simulink model "sim_flexible_unsteady_indi"  (R2018b)
settings: Solver=ode4  StartTime=0.0  StopTime=1000  FixedStep=1/600  RelTol=1e-2  AbsTol=1e-2
model workspace (MAT data in the model file):
  Var = 0
undefined symbols (not defined in the file): aircraft, gla_indi, jystck
libraries: se2a_controller_lib x2, InputBlocks_library x2, se2a_environment_lib x1, flight_dynamics_models x1, sensors_lib x1, aeroelasticity_lib x1, se2a_command_lib x1, joystick_lib x1, dspnetwork x1, flexiFlightVis_lib x1
settings Model: PacingRate=0.100000  ParamWorkspaceSource=ReferencedWorkspace  TunableVars=test_val  TunableVarsStorageClass=ExportedGlobal  Creator=Yannic  LastModifiedBy=yannic
settings DataIOCC: ExternalInput=[0,tp_indi.Input']  InitialState=tp_indi.State  LoadExternalInput=on  LoadInitialState=on
settings DebuggingCC: InitInArrayFormatMsg=none

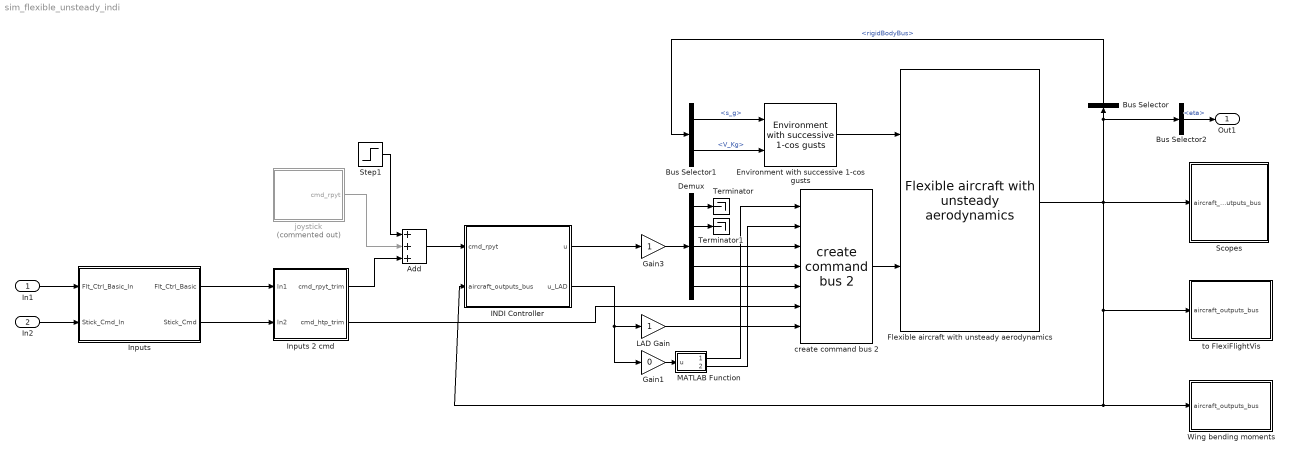
== system sim_flexible_unsteady_indi ==
  In1 : Inport
  In2 : Inport  Port=2
  Add : Sum  Inputs=+++
  Bus Selector : BusSelector  OutputSignals=flexible_body_bus.rigidBodyBus
  Bus Selector1 : BusSelector  OutputSignals=s_g,V_Kg
  Bus Selector2 : BusSelector  OutputSignals=flexible_body_bus.eta
  Demux : Demux  Outputs=5
  Environment with successive 1-cos gusts : se2a_environment_lib/Environment with successive 1-cos gusts  envir=envir  wind_input=2  F_g=1  gustGradDist=100  Delta_gustGradDist=100  Delta_time=3  time_0=1
      settings: SourceProductName=SE2A library
  Flexible aircraft with unsteady aerodynamics : flight_dynamics_models/Flexible aircraft with unsteady aerodynamics  aircraft=aircraft  ic=ic
      settings: SourceProductName=SE2A library
  Gain1 : Gain  Gain=0
  Gain3 : Gain
  INDI Controller : Subsystem
  Inputs : Subsystem
  Inputs 2 cmd : Subsystem
  LAD Gain : Gain
  MATLAB Function : MATLAB Function  TreatAsAtomicUnit=on
  Scopes : Subsystem
  Step1 : Step  Before=zeros(4,1)  After=[0;0.05;0;0]*0  SampleTime=0
  Terminator : Terminator
  Terminator1 : Terminator
  Wing bending moments : Subsystem
  create command bus 2 : se2a_command_lib/create command bus 2
      settings: SourceProductName=SE2A library
  joystick : Subsystem  Commented=on
  to FlexiFlightVis : Subsystem
  Out1 : Outport
  wires:
  Environment with successive 1-cos gusts/1 -> Flexible aircraft with unsteady aerodynamics/1
  create command bus 2/1 -> Flexible aircraft with unsteady aerodynamics/2
  Bus Selector1/1 -> Environment with successive 1-cos gusts/1  "<s_g>"
  Bus Selector/1 -> Bus Selector1/1  "<rigidBodyBus>"
  Bus Selector1/2 -> Environment with successive 1-cos gusts/2  "<V_Kg>"
  joystick/1(cmd_rpyt) -> Add/2
  Flexible aircraft with unsteady aerodynamics/1 -> to FlexiFlightVis/1(aircraft_outputs_bus), Wing bending moments/1(aircraft_outputs_bus), INDI Controller/2(aircraft_outputs_bus), Scopes/1(aircraft_outputs_bus), Bus Selector2/1, Bus Selector/1
  Demux/3 -> create command bus 2/3
  Demux/4 -> create command bus 2/4
  Demux/5 -> create command bus 2/5
  Inputs 2 cmd/2(cmd_htp_trim) -> create command bus 2/6
  In1/1 -> Inputs/1(Flt_Ctrl_Basic_In)
  In2/1 -> Inputs/2(Stick_Cmd_In)
  Inputs/1(Flt_Ctrl_Basic) -> Inputs 2 cmd/1(In1)
  Inputs/2(Stick_Cmd) -> Inputs 2 cmd/2(In2)
  Add/1 -> INDI Controller/1(cmd_rpyt)
  Inputs 2 cmd/1(cmd_rpyt_trim) -> Add/3
  INDI Controller/1(u) -> Gain3/1
  Gain3/1 -> Demux/1
  INDI Controller/2(u_LAD) -> Gain1/1, LAD Gain/1
  Step1/1 -> Add/1
  LAD Gain/1 -> create command bus 2/7
  Bus Selector2/1 -> Out1/1  "<eta>"
  Gain1/1 -> MATLAB Function/1(u)
  MATLAB Function/1(a_l) -> create command bus 2/1
  MATLAB Function/2(a_r) -> create command bus 2/2
  Demux/1 -> Terminator/1
  Demux/2 -> Terminator1/1

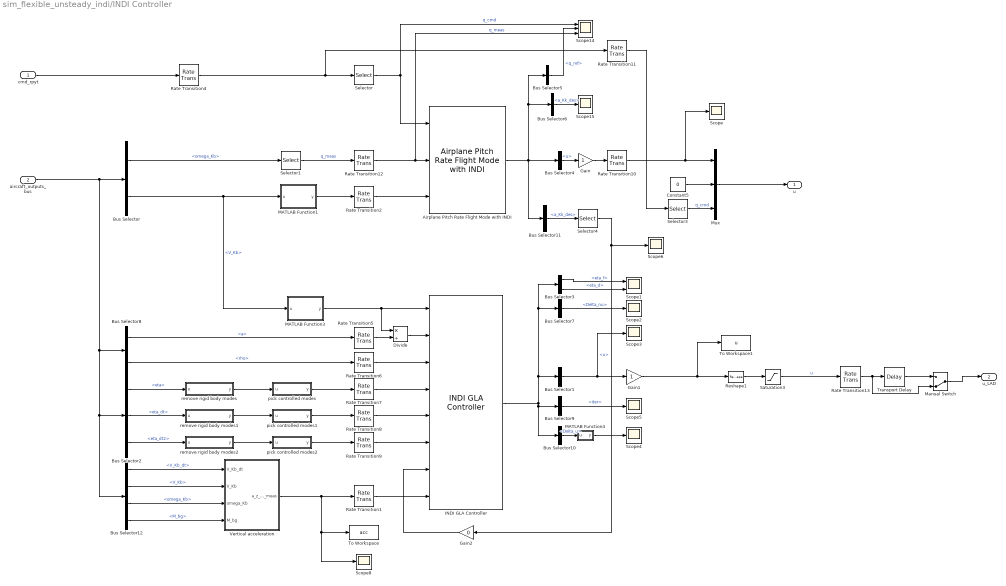
== system sim_flexible_unsteady_indi/INDI Controller ==
  cmd_rpyt : Inport
  aircraft_outputs_bus : Inport  Port=2
  Airplane Pitch Rate Flight Mode with INDI : se2a_controller_lib/Airplane Pitch Rate Flight Mode with INDI  fm=pitch_rate_controller
  Bus Selector : BusSelector  OutputSignals=flexible_body_bus.rigidBodyBus.omega_Kb,flexible_body_bus.rigidBodyBus.V_Kb
  Bus Selector1 : BusSelector  OutputSignals=u
  Bus Selector10 : BusSelector  OutputSignals=Delta_u
  Bus Selector11 : BusSelector  OutputSignals=direct_lift_control.a_Kk_des
  Bus Selector12 : BusSelector  OutputSignals=flexible_body_bus.rigidBodyBus.V_Kb_dt,flexible_body_bus.rigidBodyBus.V_Kb,flexible_body_bus.rigidBodyBus.omega_Kb,flexible_body_bus.rigidBodyBus.M_bg
  Bus Selector2 : BusSelector  OutputSignals=flexible_body_bus.eta,flexible_body_bus.eta_dt,flexible_body_bus.eta_dt2
  Bus Selector3 : BusSelector  OutputSignals=measure.eta_f,desired.eta_d
  Bus Selector4 : BusSelector  OutputSignals=u
  Bus Selector5 : BusSelector  OutputSignals=pitch_rate_control.reference.q_ref
  Bus Selector6 : BusSelector  OutputSignals=direct_lift_control.a_Kk_des
  Bus Selector7 : BusSelector  OutputSignals=pseudo_cntrl.Delta_nu
  Bus Selector8 : BusSelector  OutputSignals=aeroBus.main.external.atmosphere.a,aeroBus.main.external.atmosphere.rho
  Bus Selector9 : BusSelector  OutputSignals=iter
  Constant5 : Constant  Value=0
  Divide : Product  Inputs=*/
  Gain : Gain
  Gain1 : Gain
  Gain2 : Gain  Gain=0
  INDI GLA Controller : se2a_controller_lib/INDI GLA Controller  gla_indi=gla_indi
  MATLAB Function1 : MATLAB Function  TreatAsAtomicUnit=on
  MATLAB Function3 : MATLAB Function  TreatAsAtomicUnit=on
  MATLAB Function4 : MATLAB Function  TreatAsAtomicUnit=on
  Manual Switch : ManualSwitch  CurrentSetting=0
  Mux : Mux  Inputs=3
  Rate Transition{1,5..9} (6 alike) : RateTransition  OutPortSampleTime=gla_indi.ts
  Rate Transition{2,4,10..13} (6 alike) : RateTransition
  Reshape1 : Reshape
  Saturation3 : Saturate  UpperLimit=gla_indi.ca.u_max  LowerLimit=gla_indi.ca.u_min
  Scope{,2..6,8,15} (8 alike) : Scope
  Scope1 : Scope  NumInputPorts=2
  Scope14 : Scope  NumInputPorts=3
  Selector : Selector  InputPortWidth=4  IndexOptions=Index vector (dialog)  Indices=2  OutputSizes=1
  Selector1 : Selector  InputPortWidth=3  IndexOptions=Index vector (dialog)  Indices=2  OutputSizes=1
  Selector3 : Selector  InputPortWidth=4  IndexOptions=Index vector (dialog)  Indices=4  OutputSizes=1
  Selector4 : Selector  InputPortWidth=3  IndexOptions=Index vector (dialog)  Indices=3  OutputSizes=1
  To Workspace : ToWorkspace  VariableName=acc  SaveFormat=Timeseries  SampleTime=-1
  To Workspace1 : ToWorkspace  VariableName=u  SaveFormat=Timeseries  SampleTime=-1
  Transport Delay : TransportDelay  DelayTime=gla_indi.ts  TransDelayFeedthrough=on
  Vertical acceleration : Subsystem
  pick controlled modes : MATLAB Function  TreatAsAtomicUnit=on
  pick controlled modes1 : MATLAB Function  TreatAsAtomicUnit=on
  pick controlled modes2 : MATLAB Function  TreatAsAtomicUnit=on
  remove rigid body modes : MATLAB Function  TreatAsAtomicUnit=on
  remove rigid body modes1 : MATLAB Function  TreatAsAtomicUnit=on
  remove rigid body modes2 : MATLAB Function  TreatAsAtomicUnit=on
  u : Outport
  u_LAD : Outport  Port=2
  wires:
  cmd_rpyt/1 -> Rate Transition4/1
  aircraft_outputs_bus/1 -> Bus Selector12/1, Bus Selector2/1, Bus Selector8/1, Bus Selector/1
  Bus Selector/1 -> Selector1/1  "<omega_Kb>"
  Bus Selector/2 -> MATLAB Function3/1(u), MATLAB Function1/1(u)  "<V_Kb>"
  Rate Transition2/1 -> Airplane Pitch Rate Flight Mode with INDI/3
  Rate Transition4/1 -> Rate Transition11/1, Selector/1
  Bus Selector4/1 -> Gain/1  "<u>"
  Rate Transition10/1 -> Scope/1, Mux/1
  Constant5/1 -> Mux/2
  Bus Selector5/1 -> Scope14/2  "<q_ref>"
  Selector/1 -> Airplane Pitch Rate Flight Mode with INDI/1, Scope14/1  "q_cmd"
  Bus Selector6/1 -> Scope15/1  "<a_Kk_des>"
  Rate Transition12/1 -> Airplane Pitch Rate Flight Mode with INDI/2, Scope14/3  "q_meas"
  Airplane Pitch Rate Flight Mode with INDI/1 -> Bus Selector5/1, Bus Selector6/1, Bus Selector11/1, Bus Selector4/1
  Mux/1 -> u/1
  Bus Selector2/1 -> remove rigid body modes/1(u)  "<eta>"
  INDI GLA Controller/1 -> Bus Selector10/1, Bus Selector9/1, Bus Selector7/1, Bus Selector3/1, Bus Selector1/1
  Bus Selector2/2 -> remove rigid body modes1/1(u)  "<eta_dt>"
  Bus Selector2/3 -> remove rigid body modes2/1(u)  "<eta_dt2>"
  Bus Selector1/1 -> Scope3/1, Gain1/1  "<u>"
  Bus Selector3/1 -> Scope1/1  "<eta_f>"
  Bus Selector3/2 -> Scope1/2  "<eta_d>"
  Gain/1 -> Rate Transition10/1
  remove rigid body modes/1(y) -> pick controlled modes/1(u)
  remove rigid body modes1/1(y) -> pick controlled modes1/1(u)
  remove rigid body modes2/1(y) -> pick controlled modes2/1(u)
  Bus Selector7/1 -> Scope2/1  "<Delta_nu>"
  Bus Selector8/2 -> Rate Transition6/1  "<rho>"
  Bus Selector8/1 -> Rate Transition5/1  "<a>"
  Bus Selector9/1 -> Scope5/1  "<iter>"
  Divide/1 -> INDI GLA Controller/2
  Rate Transition5/1 -> Divide/2
  Rate Transition6/1 -> INDI GLA Controller/3
  Rate Transition7/1 -> INDI GLA Controller/4
  Rate Transition8/1 -> INDI GLA Controller/5
  Rate Transition9/1 -> INDI GLA Controller/6
  Selector3/1 -> Mux/3  "q_cmd"
  Rate Transition11/1 -> Selector3/1
  Rate Transition13/1 -> Manual Switch/2, Transport Delay/1
  Gain1/1 -> To Workspace1/1, Reshape1/1
  Transport Delay/1 -> Manual Switch/1
  Reshape1/1 -> Saturation3/1
  Bus Selector10/1 -> MATLAB Function4/1(u)  "<Delta_u>"
  MATLAB Function4/1(y) -> Scope4/1
  Saturation3/1 -> Rate Transition13/1  "u"
  Bus Selector11/1 -> Selector4/1  "<a_Kk_des>"
  Selector4/1 -> Scope6/1, Gain2/1
  pick controlled modes/1(y) -> Rate Transition7/1
  pick controlled modes1/1(y) -> Rate Transition8/1
  pick controlled modes2/1(y) -> Rate Transition9/1
  Manual Switch/1 -> u_LAD/1
  Selector1/1 -> Rate Transition12/1  "q_meas"
  MATLAB Function3/1(y) -> INDI GLA Controller/1, Divide/1
  Gain2/1 -> INDI GLA Controller/7
  MATLAB Function1/1(y) -> Rate Transition2/1
  Bus Selector12/1 -> Vertical acceleration/1(V_Kb_dt)  "<V_Kb_dt>"
  Bus Selector12/2 -> Vertical acceleration/2(V_Kb)  "<V_Kb>"
  Bus Selector12/3 -> Vertical acceleration/3(omega_Kb)  "<omega_Kb>"
  Bus Selector12/4 -> Vertical acceleration/4(M_bg)  "<M_bg>"
  Vertical acceleration/1(a_z_Kb_meas) -> Scope8/1, To Workspace/1, Rate Transition1/1
  Rate Transition1/1 -> INDI GLA Controller/8

== system sim_flexible_unsteady_indi/Inputs ==
  Flt_Ctrl_Basic_In : Inport
  Stick_Cmd_In : Inport  Port=2
  FltCtrlBasic : InputBlocks_library/FltCtrlBasic  SystemSampleTime=-1
  StickCmd : InputBlocks_library/StickCmd  SystemSampleTime=-1
  Flt_Ctrl_Basic : Outport
  Stick_Cmd : Outport  Port=2
  wires:
  StickCmd/1 -> Stick_Cmd/1
  FltCtrlBasic/1 -> Flt_Ctrl_Basic/1
  Flt_Ctrl_Basic_In/1 -> FltCtrlBasic/1
  Stick_Cmd_In/1 -> StickCmd/1

== system sim_flexible_unsteady_indi/Inputs 2 cmd ==
  In1 : Inport
  In2 : Inport  Port=2
  Demux : Demux  Outputs=2
  Mux : Mux  Inputs=2
  Selector : Selector  InputPortWidth=4  IndexOptions=Index vector (dialog)  Indices=1:3  OutputSizes=1
  cmd_rpyt_trim : Outport
  cmd_htp_trim : Outport  Port=2
  wires:
  Demux/1 -> Mux/2
  Selector/1 -> Mux/1
  Mux/1 -> cmd_rpyt_trim/1
  In1/1 -> Demux/1
  Demux/2 -> cmd_htp_trim/1
  In2/1 -> Selector/1

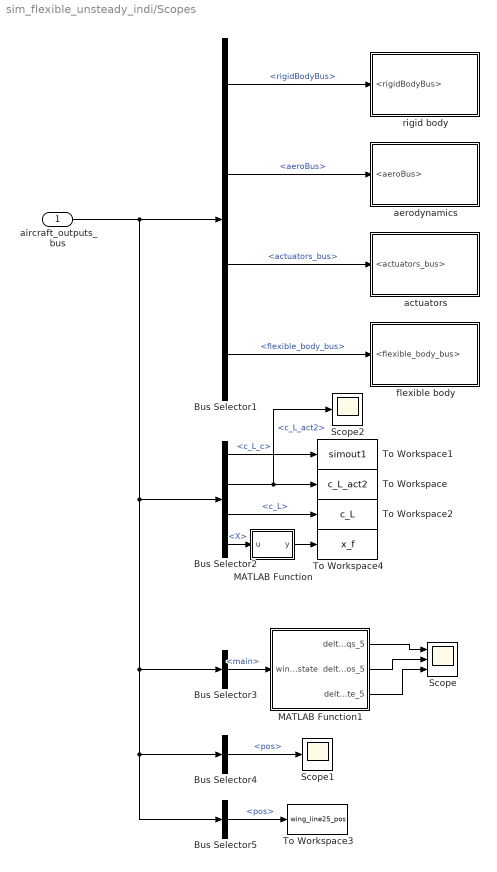
== system sim_flexible_unsteady_indi/Scopes ==
  aircraft_outputs_bus : Inport
  Bus Selector1 : BusSelector  OutputSignals=flexible_body_bus.rigidBodyBus,aeroBus,actuators_bus,flexible_body_bus
  Bus Selector2 : BusSelector  OutputSignals=aeroBus.main.aero.unsteady.c_L_c,aeroBus.main.aero.unsteady.c_L_act2,aeroBus.main.aero.circulation.c_L,aeroBus.main.aero.unsteady.X
  Bus Selector3 : BusSelector  OutputSignals=aeroBus.main
  Bus Selector4 : BusSelector  OutputSignals=aeroBus.main.actuators.pos
  Bus Selector5 : BusSelector  OutputSignals=aeroBus.main.geometry.line_25.pos
  MATLAB Function : MATLAB Function  TreatAsAtomicUnit=on
  MATLAB Function1 : MATLAB Function  TreatAsAtomicUnit=on
  Scope : Scope  NumInputPorts=3
  Scope1 : Scope
  Scope2 : Scope
  To Workspace : ToWorkspace  VariableName=c_L_act2  SaveFormat=Timeseries  SampleTime=-1
  To Workspace1 : ToWorkspace  VariableName=simout1  SaveFormat=Timeseries  SampleTime=-1
  To Workspace2 : ToWorkspace  VariableName=c_L  SaveFormat=Timeseries  SampleTime=-1
  To Workspace3 : ToWorkspace  VariableName=wing_line25_pos  SaveFormat=Timeseries  SampleTime=-1
  To Workspace4 : ToWorkspace  VariableName=x_f  SaveFormat=Timeseries  SampleTime=-1
  actuators : Subsystem
  aerodynamics : Subsystem
  flexible body : Subsystem
  rigid body : Subsystem
  wires:
  Bus Selector1/1 -> rigid body/1(<rigidBodyBus>)  "<rigidBodyBus>"
  Bus Selector1/2 -> aerodynamics/1(<aeroBus>)  "<aeroBus>"
  Bus Selector1/3 -> actuators/1(<actuators_bus>)  "<actuators_bus>"
  Bus Selector1/4 -> flexible body/1(<flexible_body_bus>)  "<flexible_body_bus>"
  MATLAB Function1/1(delta_qs_5) -> Scope/1
  MATLAB Function1/3(delta_qs_rate_5) -> Scope/3
  Bus Selector2/3 -> To Workspace2/1  "<c_L>"
  MATLAB Function1/2(delta_qs_pos_5) -> Scope/2
  Bus Selector3/1 -> MATLAB Function1/1(wing_state)  "<main>"
  Bus Selector2/2 -> Scope2/1, To Workspace/1  "<c_L_act2>"
  aircraft_outputs_bus/1 -> Bus Selector5/1, Bus Selector4/1, Bus Selector3/1, Bus Selector2/1, Bus Selector1/1
  Bus Selector2/1 -> To Workspace1/1  "<c_L_c>"
  Bus Selector4/1 -> Scope1/1  "<pos>"
  Bus Selector5/1 -> To Workspace3/1  "<pos>"
  Bus Selector2/4 -> MATLAB Function/1(u)  "<X>"
  MATLAB Function/1(y) -> To Workspace4/1

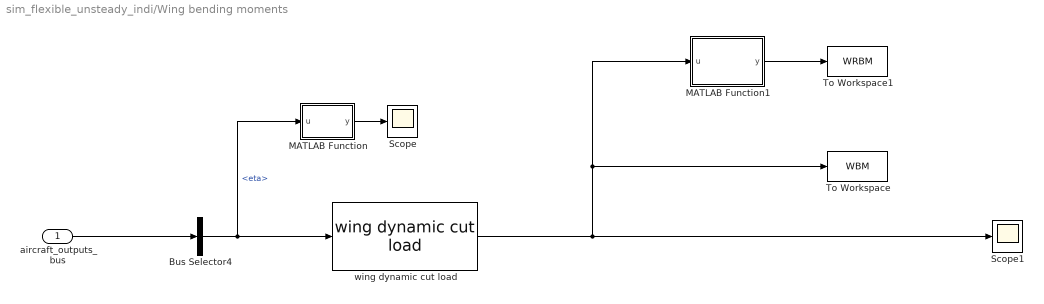
== system sim_flexible_unsteady_indi/Wing bending moments ==
  aircraft_outputs_bus : Inport
  Bus Selector4 : BusSelector  OutputSignals=flexible_body_bus.eta
  MATLAB Function : MATLAB Function  TreatAsAtomicUnit=on
  MATLAB Function1 : MATLAB Function  TreatAsAtomicUnit=on
  Scope : Scope
  Scope1 : Scope
  To Workspace : ToWorkspace  VariableName=WBM  SaveFormat=Timeseries  SampleTime=-1
  To Workspace1 : ToWorkspace  VariableName=WRBM  SaveFormat=Timeseries  SampleTime=-1
  wing dynamic cut load : aeroelasticity_lib/wing dynamic cut load  structure=structure  structure_red=aircraft.eom_flexible.structure_red  eta=[-0.9:0.2:0.9]  popup_index_1=Mx  popup_index_2=reverse_right
      settings: SourceProductName=LADAC
  wires:
  Bus Selector4/1 -> wing dynamic cut load/1, MATLAB Function/1(u)  "<eta>"
  aircraft_outputs_bus/1 -> Bus Selector4/1
  wing dynamic cut load/1 -> Scope1/1, To Workspace/1, MATLAB Function1/1(u)
  MATLAB Function/1(y) -> Scope/1
  MATLAB Function1/1(y) -> To Workspace1/1

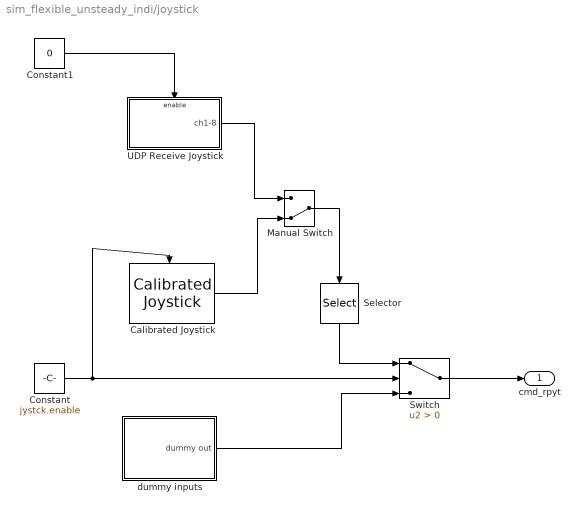
== system sim_flexible_unsteady_indi/joystick ==
  Calibrated Joystick : joystick_lib/Calibrated Joystick  jystck=jystck
      settings: SourceProductName=LADAC
  Constant : Constant  Value=jystck.enable
  Constant1 : Constant  Value=0
  Manual Switch : ManualSwitch  CurrentSetting=0
  Selector : Selector  InputPortWidth=8  IndexOptions=Index vector (dialog)  Indices=[1,2,3,4]  OutputSizes=1
  Switch : Switch  Criteria=u2 > Threshold
  UDP Receive Joystick : Subsystem
  dummy inputs : Subsystem
  cmd_rpyt : Outport
  wires:
  Switch/1 -> cmd_rpyt/1
  Constant/1 -> Calibrated Joystick/Enable, Switch/2
  dummy inputs/1(dummy out) -> Switch/3
  Selector/1 -> Switch/1
  UDP Receive Joystick/1(ch1-8) -> Manual Switch/1
  Manual Switch/1 -> Selector/1
  Calibrated Joystick/1 -> Manual Switch/2
  Constant1/1 -> UDP Receive Joystick/Enable

== system sim_flexible_unsteady_indi/to FlexiFlightVis ==
  aircraft_outputs_bus : Inport
  Bus Creator : BusCreator  Inputs=1
  Bus Selector : BusSelector  OutputSignals=flexible_body_bus.rigidBodyBus,aeroBus.main,aeroBus.htp,aeroBus.vtp,aeroBus.fuselage
  Constant : Constant  Value=aircraft.config.xyz_ref_c
  Send to FlexiFlightVis : flexiFlightVis_lib/Send to FlexiFlightVis  sample_time=1/60  ip_address='localhost'  ip_port=4321  wing_cell={aircraft.wing_main.state,aircraft.wing_htp.state,aircraft.wing_vtp.state}  fuse_cell={aircraft.fuselage.state}
      settings: SourceProductName=LADAC
  wires:
  aircraft_outputs_bus/1 -> Bus Selector/1
  Bus Selector/4 -> Send to FlexiFlightVis/5  "<vtp>"
  Bus Selector/5 -> Send to FlexiFlightVis/6  "<fuselage>"
  Bus Selector/3 -> Send to FlexiFlightVis/4  "<htp>"
  Bus Selector/2 -> Send to FlexiFlightVis/3  "<main>"
  Bus Selector/1 -> Send to FlexiFlightVis/1  "<rigidBodyBus>"
  Constant/1 -> Bus Creator/1  "xyz_ref_c"
  Bus Creator/1 -> Send to FlexiFlightVis/2

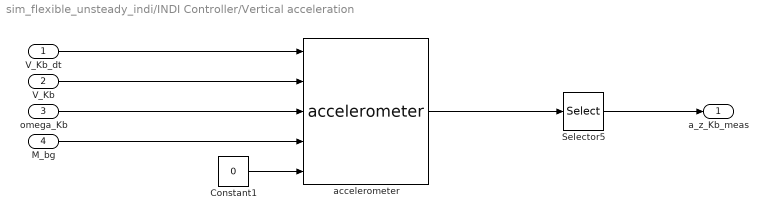
== system sim_flexible_unsteady_indi/INDI Controller/Vertical acceleration ==
  V_Kb_dt : Inport
  V_Kb : Inport  Port=2
  omega_Kb : Inport  Port=3
  M_bg : Inport  Port=4
  Constant1 : Constant  Value=0  VectorParams1D=off
  Selector5 : Selector  InputPortWidth=3  IndexOptions=Index vector (dialog)  Indices=3  OutputSizes=1
  accelerometer : sensors_lib/accelerometer  SystemSampleTime=-1
      settings: SourceProductName=LADAC
  a_z_Kb_meas : Outport
  wires:
  M_bg/1 -> accelerometer/4
  Selector5/1 -> a_z_Kb_meas/1
  accelerometer/1 -> Selector5/1
  V_Kb/1 -> accelerometer/2
  omega_Kb/1 -> accelerometer/3
  V_Kb_dt/1 -> accelerometer/1
  Constant1/1 -> accelerometer/5

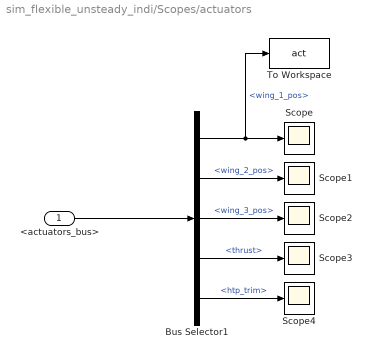
== system sim_flexible_unsteady_indi/Scopes/actuators ==
  <actuators_bus> : Inport
  Bus Selector1 : BusSelector  OutputSignals=wing_1_pos,wing_2_pos,wing_3_pos,thrust,htp_trim
  Scope{,1..4} (5 alike) : Scope
  To Workspace : ToWorkspace  VariableName=act  SaveFormat=Timeseries  SampleTime=-1
  wires:
  <actuators_bus>/1 -> Bus Selector1/1
  Bus Selector1/1 -> To Workspace/1, Scope/1  "<wing_1_pos>"
  Bus Selector1/2 -> Scope1/1  "<wing_2_pos>"
  Bus Selector1/3 -> Scope2/1  "<wing_3_pos>"
  Bus Selector1/4 -> Scope3/1  "<thrust>"
  Bus Selector1/5 -> Scope4/1  "<htp_trim>"

== system sim_flexible_unsteady_indi/Scopes/aerodynamics ==
  <aeroBus> : Inport
  Bus Selector1 : BusSelector  OutputSignals=main,htp,vtp
  htp : Subsystem
  vtp : Subsystem
  wing : Subsystem
  wires:
  <aeroBus>/1 -> Bus Selector1/1
  Bus Selector1/2 -> htp/1(htp)  "<htp>"
  Bus Selector1/1 -> wing/1(main)  "<main>"
  Bus Selector1/3 -> vtp/1(vtp)  "<vtp>"

== system sim_flexible_unsteady_indi/Scopes/flexible body ==
  <flexible_body_bus> : Inport
  Bus Selector1 : BusSelector  OutputSignals=eta,eta_dt,eta_dt2,generalized_load_vector
  Scope{,1..3} (4 alike) : Scope
  To Workspace : ToWorkspace  VariableName=eta  SaveFormat=Timeseries  SampleTime=-1
  wires:
  Bus Selector1/4 -> Scope3/1  "<generalized_load_vector>"
  Bus Selector1/3 -> Scope2/1  "<eta_dt2>"
  Bus Selector1/2 -> Scope1/1  "<eta_dt>"
  Bus Selector1/1 -> To Workspace/1, Scope/1  "<eta>"
  <flexible_body_bus>/1 -> Bus Selector1/1

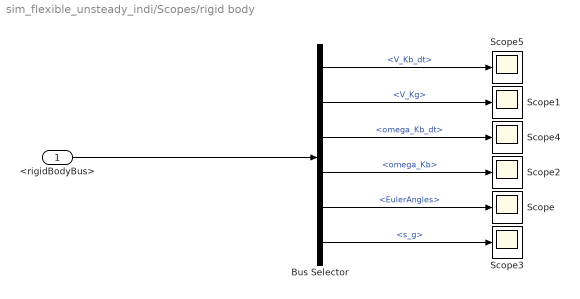
== system sim_flexible_unsteady_indi/Scopes/rigid body ==
  <rigidBodyBus> : Inport
  Bus Selector : BusSelector  OutputSignals=V_Kb_dt,V_Kg,omega_Kb_dt,omega_Kb,EulerAngles,s_g
  Scope{,1..5} (6 alike) : Scope
  wires:
  Bus Selector/5 -> Scope/1  "<EulerAngles>"
  Bus Selector/2 -> Scope1/1  "<V_Kg>"
  Bus Selector/6 -> Scope3/1  "<s_g>"
  Bus Selector/4 -> Scope2/1  "<omega_Kb>"
  <rigidBodyBus>/1 -> Bus Selector/1
  Bus Selector/3 -> Scope4/1  "<omega_Kb_dt>"
  Bus Selector/1 -> Scope5/1  "<V_Kb_dt>"

== system sim_flexible_unsteady_indi/joystick/UDP Receive Joystick ==
  Enable : EnablePort
  Terminator : Terminator
  UDP Receive1 : dspnetwork/UDP Receive  localURL='0.0.0.0'  localPort=25000  remoteURL='192.168.178.2'  remotePort=-1  recvBufferSize=8*8  dims=8  signalDatatype=double  isVarSize=off  showBlockingTime=on  blockingTime=1  sampletime=1/30  blockPlatform=HOST
      settings: SourceProductName=DSP System Toolbox  SourceProductBaseCode=DS
  ch1-8 : Outport
  wires:
  UDP Receive1/1 -> ch1-8/1
  UDP Receive1/2 -> Terminator/1

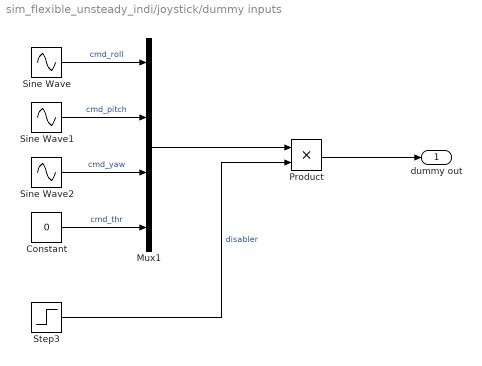
== system sim_flexible_unsteady_indi/joystick/dummy inputs ==
  Constant : Constant  Value=0
  Mux1 : Mux
  Product : Product
  Sine Wave : Sin  Amplitude=0.1  Frequency=3  SampleTime=0
  Sine Wave1 : Sin  Amplitude=0.1  Frequency=4  SampleTime=0
  Sine Wave2 : Sin  Amplitude=0.1  Frequency=5  SampleTime=0
  Step3 : Step  Time=10  Before=1  After=0  SampleTime=0
  dummy out : Outport
  wires:
  Constant/1 -> Mux1/4  "cmd_thr"
  Sine Wave2/1 -> Mux1/3  "cmd_yaw"
  Sine Wave1/1 -> Mux1/2  "cmd_pitch"
  Sine Wave/1 -> Mux1/1  "cmd_roll"
  Mux1/1 -> Product/1
  Product/1 -> dummy out/1
  Step3/1 -> Product/2  "disabler"

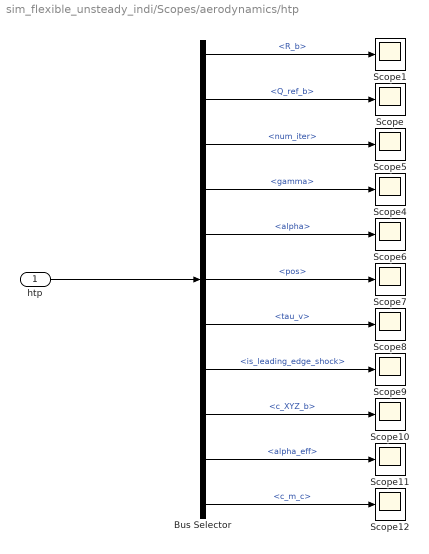
== system sim_flexible_unsteady_indi/Scopes/aerodynamics/htp ==
  htp : Inport
  Bus Selector : BusSelector  OutputSignals=aero.force_glob.R_b,aero.force_glob.Q_ref_b,aero.circulation.num_iter,aero.circulation.gamma,body.alpha,actuators.pos,aero.unsteady.tau_v,aero.unsteady.is_leading_edge_shock,aero.coeff_loc.c_XYZ_b,aero.circulation.alpha_eff,aero.unsteady.c_m_c
  Scope{,1,4..12} (11 alike) : Scope
  wires:
  Bus Selector/11 -> Scope12/1  "<c_m_c>"
  Bus Selector/10 -> Scope11/1  "<alpha_eff>"
  Bus Selector/9 -> Scope10/1  "<c_XYZ_b>"
  Bus Selector/8 -> Scope9/1  "<is_leading_edge_shock>"
  Bus Selector/7 -> Scope8/1  "<tau_v>"
  Bus Selector/6 -> Scope7/1  "<pos>"
  Bus Selector/5 -> Scope6/1  "<alpha>"
  htp/1 -> Bus Selector/1
  Bus Selector/1 -> Scope1/1  "<R_b>"
  Bus Selector/2 -> Scope/1  "<Q_ref_b>"
  Bus Selector/4 -> Scope4/1  "<gamma>"
  Bus Selector/3 -> Scope5/1  "<num_iter>"

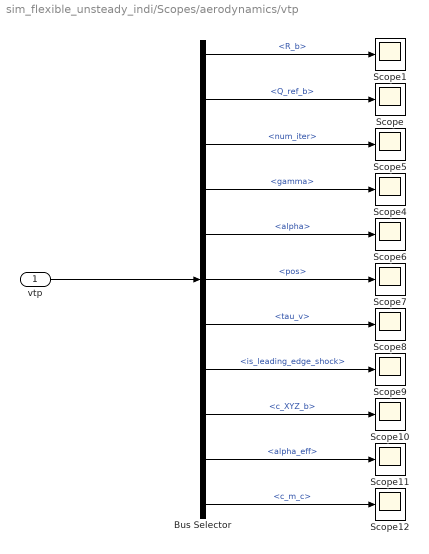
== system sim_flexible_unsteady_indi/Scopes/aerodynamics/vtp ==
  vtp : Inport
  Bus Selector : BusSelector  OutputSignals=aero.force_glob.R_b,aero.force_glob.Q_ref_b,aero.circulation.num_iter,aero.circulation.gamma,body.alpha,actuators.pos,aero.unsteady.tau_v,aero.unsteady.is_leading_edge_shock,aero.coeff_loc.c_XYZ_b,aero.circulation.alpha_eff,aero.unsteady.c_m_c
  Scope{,1,4..12} (11 alike) : Scope
  wires:
  Bus Selector/3 -> Scope5/1  "<num_iter>"
  Bus Selector/4 -> Scope4/1  "<gamma>"
  Bus Selector/2 -> Scope/1  "<Q_ref_b>"
  Bus Selector/1 -> Scope1/1  "<R_b>"
  vtp/1 -> Bus Selector/1
  Bus Selector/5 -> Scope6/1  "<alpha>"
  Bus Selector/6 -> Scope7/1  "<pos>"
  Bus Selector/7 -> Scope8/1  "<tau_v>"
  Bus Selector/8 -> Scope9/1  "<is_leading_edge_shock>"
  Bus Selector/9 -> Scope10/1  "<c_XYZ_b>"
  Bus Selector/10 -> Scope11/1  "<alpha_eff>"
  Bus Selector/11 -> Scope12/1  "<c_m_c>"

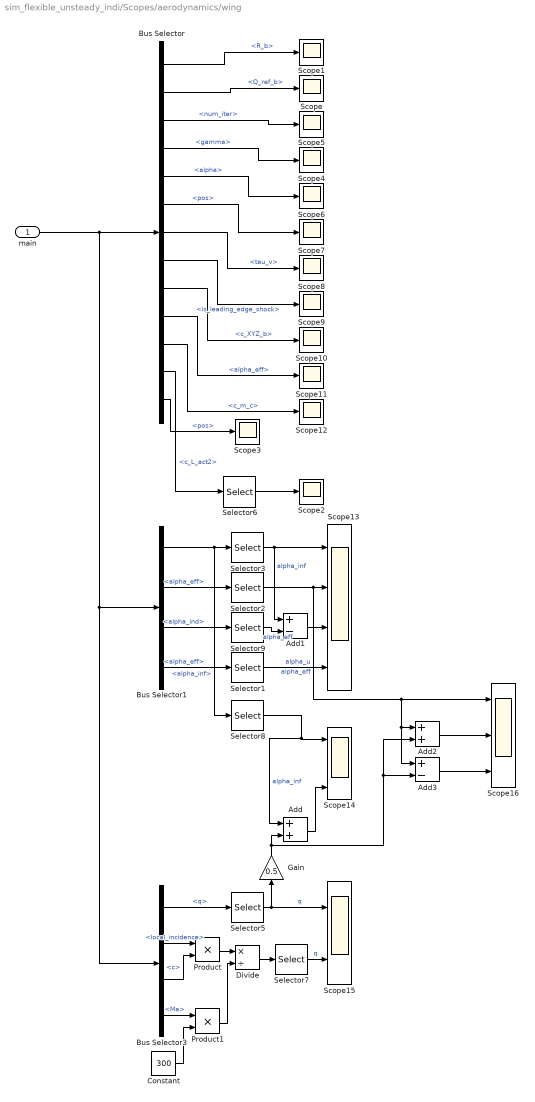
== system sim_flexible_unsteady_indi/Scopes/aerodynamics/wing ==
  main : Inport
  Add : Sum
  Add1 : Sum  Inputs=+-
  Add2 : Sum
  Add3 : Sum  Inputs=+-
  Bus Selector : BusSelector  OutputSignals=aero.force_glob.R_b,aero.force_glob.Q_ref_b,aero.circulation.num_iter,aero.circulation.gamma,body.alpha,actuators.pos,aero.unsteady.tau_v,aero.unsteady.is_leading_edge_shock,aero.coeff_loc.c_XYZ_b,aero.circulation.alpha_eff,aero.unsteady.c_m_c,aero.unsteady.c_L_act2,actuators.pos
  Bus Selector1 : BusSelector  OutputSignals=aero.circulation.alpha_inf,aero.circulation.alpha_eff,aero.circulation.alpha_ind,aero.unsteady.alpha_eff
  Bus Selector3 : BusSelector  OutputSignals=aero.circulation.q,geometry.ctrl_pt_dt.local_incidence,geometry.ctrl_pt.c,aero.circulation.Ma
  Constant : Constant  Value=300
  Divide : Product  Inputs=*/
  Gain : Gain  Gain=0.5
  Product : Product
  Product1 : Product
  Scope{,1..12} (13 alike) : Scope
  Scope13 : Scope  NumInputPorts=4
  Scope14 : Scope  NumInputPorts=3
  Scope15 : Scope  NumInputPorts=2
  Scope16 : Scope  NumInputPorts=3
  Selector{1..3,5,7..9} (7 alike) : Selector  InputPortWidth=40  IndexOptions=Index vector (dialog)  Indices=1:2:9  OutputSizes=1
  Selector6 : Selector  InputPortWidth=40  IndexOptions=Index vector (dialog)  Indices=1:20  OutputSizes=1
  wires:
  Bus Selector/3 -> Scope5/1  "<num_iter>"
  Bus Selector/4 -> Scope4/1  "<gamma>"
  Bus Selector/2 -> Scope/1  "<Q_ref_b>"
  Bus Selector/1 -> Scope1/1  "<R_b>"
  main/1 -> Bus Selector3/1, Bus Selector1/1, Bus Selector/1
  Bus Selector/5 -> Scope6/1  "<alpha>"
  Bus Selector/6 -> Scope7/1  "<pos>"
  Bus Selector/7 -> Scope8/1  "<tau_v>"
  Bus Selector/8 -> Scope9/1  "<is_leading_edge_shock>"
  Bus Selector/9 -> Scope10/1  "<c_XYZ_b>"
  Bus Selector/10 -> Scope11/1  "<alpha_eff>"
  Bus Selector/11 -> Scope12/1  "<c_m_c>"
  Selector6/1 -> Scope2/1
  Bus Selector/12 -> Selector6/1  "<c_L_act2>"
  Bus Selector/13 -> Scope3/1  "<pos>"
  Bus Selector1/1 -> Selector3/1, Selector8/1  "<alpha_inf>"
  Bus Selector1/2 -> Selector2/1  "<alpha_eff>"
  Bus Selector1/4 -> Selector1/1  "<alpha_eff>"
  Selector3/1 -> Add1/1, Scope13/1  "alpha_inf"
  Selector2/1 -> Add3/1, Add2/1, Scope16/1, Scope13/2  "alpha_eff"
  Selector1/1 -> Scope13/4  "alpha_u"
  Bus Selector3/1 -> Selector5/1  "<q>"
  Selector5/1 -> Gain/1, Scope15/1  "q"
  Bus Selector3/2 -> Product/1  "<local_incidence>"
  Bus Selector3/3 -> Product/2  "<c>"
  Product/1 -> Divide/1
  Bus Selector3/4 -> Product1/1  "<Ma>"
  Constant/1 -> Product1/2
  Product1/1 -> Divide/2
  Divide/1 -> Selector7/1
  Selector7/1 -> Scope15/2  "q"
  Gain/1 -> Add2/2, Add3/2, Add/2
  Add/1 -> Scope14/3
  Selector8/1 -> Add/1, Scope14/1  "alpha_inf"
  Bus Selector1/3 -> Selector9/1  "<alpha_ind>"
  Selector9/1 -> Add1/2  "alpha_eff"
  Add1/1 -> Scope13/3
  Add2/1 -> Scope16/2
  Add3/1 -> Scope16/3

== matlab function sim_flexible_unsteady_indi/INDI Controller/pick controlled modes1 ==
  data: u input; y output; gla_indi parameter
function y = fcn(u,gla_indi)
y = u(gla_indi.mcidx);
end

== matlab function sim_flexible_unsteady_indi/INDI Controller/MATLAB Function3 ==
  data: u input; y output
function y = fcn(u)
y=norm(u,2);
end

== matlab function sim_flexible_unsteady_indi/INDI Controller/pick controlled modes2 ==
  data: u input; y output; gla_indi parameter
function y = fcn(u,gla_indi)
y = u(gla_indi.mcidx);
end

== matlab function sim_flexible_unsteady_indi/Scopes/MATLAB Function1 ==
  data: wing_state input; delta_qs_5 output; delta_qs_pos_5 output; delta_qs_rate_5 output
function [delta_qs_5,delta_qs_pos_5,delta_qs_rate_5] = fcn(wing_state)

abs_V_i = vecnorm(wing_state.aero.local_inflow.V_25,2,1);
F = airfoilFlapEffectiveness(wing_state.geometry.segments.flap_depth);
delta_qs = airfoilFlapDeltaQs( F.F_10, F.F_11,...
    abs_V_i, sum(wing_state.geometry.ctrl_pt.c,3), deg2rad(wing_state.actuators.segments.pos(2,:)), ...
    deg2rad(wing_state.actuators.segments.rate(2,:)) ) .* cos(wing_state.geometry.segments.flap_sweep);
delta_qs_pos = airfoilFlapDeltaQs( F.F_10, F.F_11,...
    abs_V_i, sum(wing_state.geometry.ctrl_pt.c,3), deg2rad(wing_state.actuators.segments.pos(2,:)), ...
    0 ) .* cos(wing_state.geometry.segments.flap_sweep);
delta_qs_rate = airfoilFlapDeltaQs( F.F_10, F.F_11,...
    abs_V_i, sum(wing_state.geometry.ctrl_pt.c,3), 0, ...
    deg2rad(wing_state.actuators.segments.rate(2,:)) ) .* cos(wing_state.geometry.segments.flap_sweep);

delta_qs_5 = delta_qs(15:19);
delta_qs_pos_5 = delta_qs_pos(15:19);
delta_qs_rate_5 = delta_qs_rate(15:19);


end

== matlab function sim_flexible_unsteady_indi/INDI Controller/remove rigid body modes ==
  data: u input; y output
function y = fcn(u)
y = u(7:end);
end

== matlab function sim_flexible_unsteady_indi/INDI Controller/remove rigid body modes1 ==
  data: u input; y output
function y = fcn(u)
y = u(7:end);
end

== matlab function sim_flexible_unsteady_indi/INDI Controller/MATLAB Function1 ==
  data: u input; y output
function y = fcn(u)
y = norm(u,2);
end

== matlab function sim_flexible_unsteady_indi/INDI Controller/remove rigid body modes2 ==
  data: u input; y output
function y = fcn(u)
y = u(7:end);
end

== matlab function sim_flexible_unsteady_indi/Wing bending moments/MATLAB Function ==
  data: u input; y output
function y = fcn(u)

y = u(7:end);

== matlab function sim_flexible_unsteady_indi/Scopes/MATLAB Function ==
  data: u input; y output
function y = fcn(u)
y = u(2,:);
end

== matlab function sim_flexible_unsteady_indi/INDI Controller/pick controlled modes ==
  data: u input; y output; gla_indi parameter
function y = fcn(u,gla_indi)
y = u(gla_indi.mcidx);
end

== matlab function sim_flexible_unsteady_indi/MATLAB Function ==
  data: u input; a_l output; a_r output
function [a_l,a_r] = fcn(u)
n_u = length(u);
a_l = u(1:n_u/2);
a_r = u(n_u/2+1:end);
end

== matlab function sim_flexible_unsteady_indi/INDI Controller/MATLAB Function4 ==
  data: u input; y output
function y = fcn(u)

y = u(10);

== matlab function sim_flexible_unsteady_indi/Wing bending moments/MATLAB Function1 ==
  data: u input; y output
function y = fcn(u)
len_u = length(u);
idx = len_u/2;
y = u([idx,idx+1]);
end
